simulink model "rtwdemo_scalarrep"  (Simulink 7.6)
settings: Solver=FixedStepDiscrete  StartTime=0.0  StopTime=10  FixedStep=.1  RelTol=1e-3
libraries: rtwdemowidgets x2
Description:
  | Optimized Vector Operations
settings Model: Creator=The MathWorks Inc.  ExtModeAutoUpdateStatusClock=off
settings MATStruct: SampleTime=.1  Offset=0  Priority=[20.0]
settings DataIOCC: SaveOutput=off  SaveTime=off
settings OptimizationCC: InlineParams=on  InlineInvariantSignals=on  StateBitsets=on  DataBitsets=on  UseTempVars=on  EfficientFloat2IntCast=on  EfficientMapNaN2IntZero=off
settings DebuggingCC: SolverPrmCheckMsg=none  StrictBusMsg=ErrorOnBusTreatedAsVector
settings HardwareCC: ProdIntDivRoundTo=Zero  ProdEndianess=LittleEndian  ProdHWDeviceType=Generic->32-bit Embedded Processor  TargetHWDeviceType=Generic->32-bit Embedded Processor
settings RTWCC: GenerateReport=on  RTWVerbose=off  ProcessScript=grt_make_rtw_hook  LaunchReport=on
settings CodeAppCC: ForceParamTrailComments=on
settings GRTTargetCC: TargetFcnLib=ansi_tfl_tmw.mat

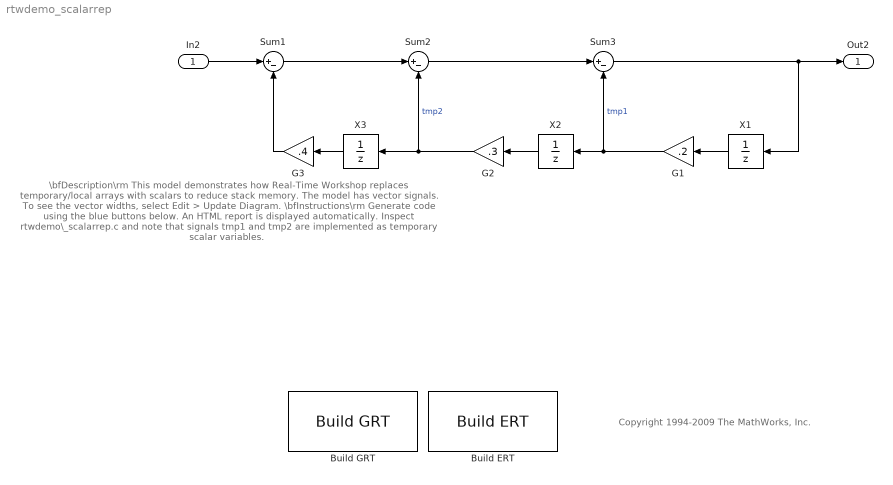
== system rtwdemo_scalarrep ==
  note: \bfDescription\rm
      | This model demonstrates how Real-Time Workshop replaces temporary/local arrays with
      | scalars to reduce stack memory. The model has vector signals. To see the vector widths,
      | select Edit > Update Diagram.
      |
      | \bfInstructions\rm
      | Generate code using the blue buttons below.  An HTML report is displayed automatically.
      | Inspect rtwdemo\_scalarrep.c and note that signals tmp1 and tmp2 are implemented as
      | temporary scalar variables.
  note: Copyright 1994-2009 The MathWorks, Inc.
  In2 : Inport  OutDataTypeStr=double  PortDimensions=10  SampleTime=.1
  Build ERT : rtwdemowidgets/Build ERT  SystemSampleTime=-1  attrib_overrides={}
  Build GRT : rtwdemowidgets/Build GRT  SystemSampleTime=-1  attrib_overrides={}
  G1 : Gain  Gain=.2
  G2 : Gain  Gain=.3
  G3 : Gain  Gain=.4
  Sum1 : Sum  Inputs=|+-
  Sum2 : Sum  Inputs=|+-
  Sum3 : Sum  Inputs=|+-
  X1 : UnitDelay  SampleTime=-1
      settings: AttributesFormatString=%<StateIdentifier>
  X2 : UnitDelay  SampleTime=-1
      settings: AttributesFormatString=%<StateIdentifier>
  X3 : UnitDelay  SampleTime=-1
      settings: AttributesFormatString=%<StateIdentifier>
  Out2 : Outport
  wires:
  In2/1 -> Sum1/1
  Sum1/1 -> Sum2/1
  Sum3/1 -> Out2/1, X1/1
  Sum2/1 -> Sum3/1
  X2/1 -> G2/1
  X1/1 -> G1/1
  G1/1 -> X2/1, Sum3/2  "tmp1"
  G2/1 -> X3/1, Sum2/2  "tmp2"
  X3/1 -> G3/1
  G3/1 -> Sum1/2
